simulink model "platform"  (Simulink 7.9)
settings: Solver=FixedStepDiscrete  StartTime=0.0  StopTime=t(end)  RelTol=1e-3
values from neighbouring files (symbols this model uses):
  Ts = C.Ts    [simulate_cl_linear.m]
undefined symbols (not defined in the file or in its folder): C
libraries: cstblocks x3
settings Model: Creator=marco  LastModifiedBy=marco
settings GRTTargetCC: CombineOutputUpdateFcns=off  GRTInterface=on

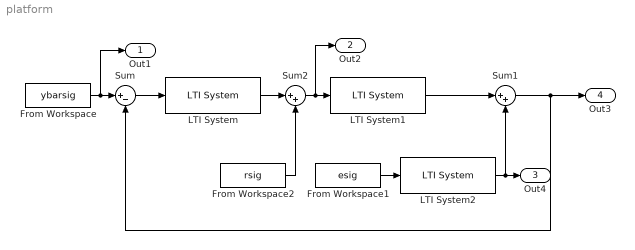
== system platform ==
  From Workspace : FromWorkspace  VariableName=ybarsig  SampleTime=Ts
  From Workspace1 : FromWorkspace  VariableName=esig  SampleTime=Ts
  From Workspace2 : FromWorkspace  VariableName=rsig  SampleTime=Ts
  LTI System : cstblocks/LTI System  sys=C  IC=zeros(size(C.A,1),1)
  LTI System1 : cstblocks/LTI System  sys=G  IC=[]
  LTI System2 : cstblocks/LTI System  sys=H  IC=[]
  Sum : Sum  Inputs=|+-
  Sum1 : Sum  Inputs=|++
  Sum2 : Sum  Inputs=|++
  Out1 : Outport
  Out2 : Outport  Port=2
  Out4 : Outport  Port=3
  Out3 : Outport  Port=4
  wires:
  Sum/1 -> LTI System/1
  LTI System1/1 -> Sum1/1
  LTI System2/1 -> Sum1/2, Out4/1
  Sum1/1 -> Sum/2, Out3/1
  From Workspace/1 -> Sum/1, Out1/1
  From Workspace1/1 -> LTI System2/1
  LTI System/1 -> Sum2/1
  Sum2/1 -> LTI System1/1, Out2/1
  From Workspace2/1 -> Sum2/2
